simulink model "downsampk8"  (R2018a)
settings: Solver=VariableStepAuto  StartTime=0.0  StopTime=10.0  RelTol=1e-3
libraries: dspsnks4 x1, dspvision x1
settings Model: Creator=ja_ping  LastModifiedBy=ja_ping

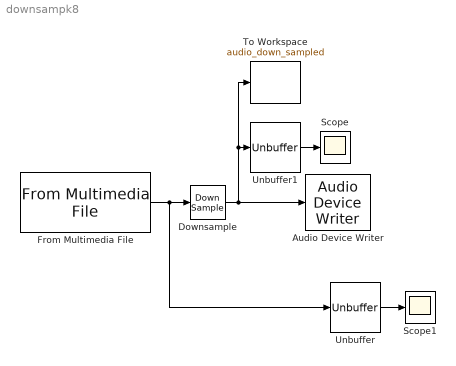
== system downsampk8 ==
  Audio Device Writer : dspsnks4/Audio Device Writer  Driver=DirectSound  Device=Default  InheritSampleRate=on  SampleRate=44100  BitDepth=16-bit integer  BufferSize=4096  NumBuffers=10  DefaultOutputChannelMapping=on  OutputChannelMapping=1:2  OutputNumUnderrunSamples=off  DriverIdx=1  DeviceWarnFlag=''
  Downsample : DownSample  N=8
  From Multimedia File : dspvision/From Multimedia File  inputFilename=G:\My Documents\MATLAB\ELEC342_lab_5_Audio.wav  loop=on  numPlays=inf  outputStreams=Audio only  videoDataType=single  audioDataType=double  inheritSampleTime=on  userDefinedSampleTime=1/30  noAudioOutput=off  isIntensityVideo=off  fourcc=RGB  colorVideoFormat=Separate color signals  outputEOF=off  dataOrg=Column-major  audioFrameSize=1024  computeAudioFrameSize=off  outSamplingMode=Sample based
      settings: SourceProductBaseCode=VP
  Scope : Scope
  Scope1 : Scope
  To Workspace : ToWorkspace  VariableName=audio_down_sampled  SampleTime=-1
      settings: MaxDataPoints=327680  Save2DSignal=2-D array (concatenate along first dimension)
  Unbuffer : Unbuffer
  Unbuffer1 : Unbuffer
  wires:
  Unbuffer1/1 -> Scope/1
  Unbuffer/1 -> Scope1/1
  From Multimedia File/1 -> Unbuffer/1, Downsample/1
  Downsample/1 -> To Workspace/1, Unbuffer1/1, Audio Device Writer/1
